simulink model "MicroMouse_RapidDevelopment"  (R2025a)
settings: Solver=FixedStepAuto  StartTime=0.0  StopTime=inf  RelTol=1e-3
PreLoadFcn:
  | addpath(genpath(pwd))
InitFcn:
  | addpath(genpath(pwd));
  | auto_program("MicroMouseProgramming_Code\build\release\MicroMouseProgramming")
  | STLINK_COMPORT = auto_COMPORT()
  | 
  | clearvars -except STLINK_COMPORT STLINK_DRIVE STM32_ODR
libraries: etargetslib x18, instrumentseriallib x2
settings Model: SILPILModeSetting=veronly  PacingRate=0.100000  ExtModeTrigDuration=10  Creator=JesseJabezArendse  LastModifiedBy=sanjannaidoo
settings SolverCC: ZeroCrossControl=EnableAll  EnableFixedStepZeroCrossing=on
settings OptimizationCC: ReuseModelBlockBuffer=off  PassReuseOutputArgsAs=Individual arguments  ZeroExternalMemoryAtStartup=off  ZeroInternalMemoryAtStartup=off  MaxStackSize=64  OptimizationLevel=level1  OptimizationCustomize=off  EfficientTunableParamExpr=on
settings DebuggingCC: SignalInfNanChecking=warning  ParameterPrecisionLossMsg=none  ParameterTunabilityLossMsg=error
settings HardwareCC: ProdBitPerPointer=32.0  ProdBitPerSizeT=32.0  ProdBitPerPtrDiffT=32.0  ProdLargestAtomicInteger=Long  ProdLargestAtomicFloat=Double  ProdWordSize=32.0  ProdLongLongMode=on  ProdHWDeviceType=ARM Compatible->ARM Cortex
settings ModelReferenceCC: EnableParallelModelReferenceBuilds=on
settings SFSimCC: SimParseCustomCode=off  MATLABDynamicMemAlloc=off  SimHardwareAcceleration=native
settings RTWCC: SystemTargetFile=ert.tlc  TemplateMakefile=ert_default_tmf  RTWUseSimCustomCode=on  Toolchain=GNU Tools for ARM Embedded Processors  BuildConfiguration=Specify  GPUComputeCapability=3.5  Description=Embedded Coder
settings CodeAppCC: ForceParamTrailComments=on  IgnoreCustomStorageClasses=off  OperatorAnnotations=on  SimulinkDataObjDesc=on  SFDataObjDesc=on  InsertBlockDesc=on
settings ERTTargetCC: ExtModeTransport=3.0  ExtModeStaticAllocSize=2000.0  InlinedParameterPlacement=Hierarchical  ERTCustomFileTemplate=example_file_process.tlc  DynamicArrayContainerType=coder::array  CodeReplacementLibrary=ARM Cortex-M  SupportContinuousTime=on
settings SimscapeCC: SimscapeLogDecimation=1  SimscapeLogDataHistory=5000

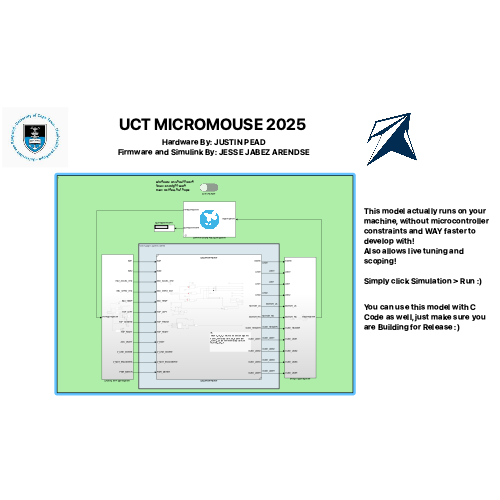
[thumbnail: Simulink's stored preview of the top-level diagram]
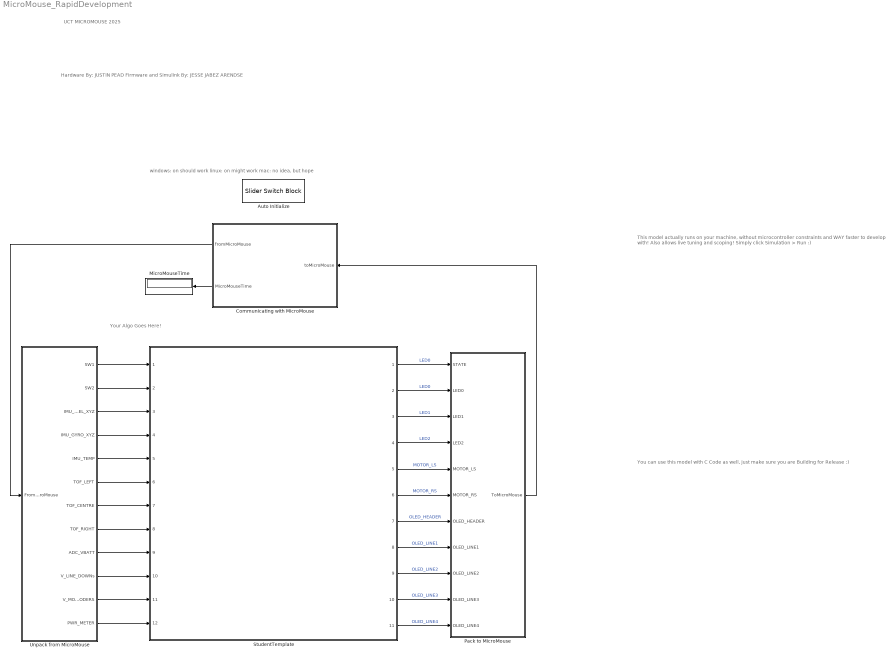
== system MicroMouse_RapidDevelopment ==
  note: windows: on should work
      | linux: on might work
      | mac: no idea, but hope
  note: Your Algo Goes Here!
  note: Hardware By: JUSTIN PEAD
      | Firmware and Simulink By: JESSE JABEZ ARENDSE
  note: UCT MICROMOUSE 2025
  note: This model actually runs on your machine, without microcontroller constraints and WAY faster to develop with!
      | Also allows live tuning and scoping!
      |
      | Simply click Simulation > Run :)
  note: You can use this model with C Code as well, just make sure you are Building for Release :)
  Auto Initialize : SliderSwitchBlock  LabelPosition=Hide
  Communicating with MicroMouse : Subsystem  mask{Auto_Initialize=0}
      mask prompts: Auto_Initialize "Automate Initialization?"
      mask TypeOptions Auto_Initialize: 1 | 0
      mask DialogControl Control1 Prompt: Block for communication between host machine and STM32L476 onboard MicroMouse
      mask Display: image('stm32_icon.png', [0,0,0,0,80,80]);
  MicroMouseTime : Display
      settings: Decimation=2
  Pack to MicroMouse : Subsystem
  StudentTemplate : Subsystem  ReferencedSubsystem=StudentTemplate
  Unpack from MicroMouse : Subsystem
  wires:
  Communicating with MicroMouse/2(MicroMouseTime) -> MicroMouseTime/1
  Pack to MicroMouse/1(ToMicroMouse) -> Communicating with MicroMouse/1(toMicroMouse)
  Communicating with MicroMouse/1(fromMicroMouse) -> Unpack from MicroMouse/1(FromMicroMouse)
  Unpack from MicroMouse/1(SW1) -> StudentTemplate/1
  Unpack from MicroMouse/2(SW2) -> StudentTemplate/2
  Unpack from MicroMouse/3(IMU_ACCEL_XYZ) -> StudentTemplate/3
  Unpack from MicroMouse/4(IMU_GYRO_XYZ) -> StudentTemplate/4
  Unpack from MicroMouse/5(IMU_TEMP) -> StudentTemplate/5
  Unpack from MicroMouse/6(TOF_LEFT) -> StudentTemplate/6
  Unpack from MicroMouse/7(TOF_CENTRE) -> StudentTemplate/7
  Unpack from MicroMouse/8(TOF_RIGHT) -> StudentTemplate/8
  Unpack from MicroMouse/9(ADC_VBATT) -> StudentTemplate/9
  Unpack from MicroMouse/10(V_LINE_DOWNs) -> StudentTemplate/10
  Unpack from MicroMouse/11(V_MOT_ENCODERS) -> StudentTemplate/11
  StudentTemplate/2 -> Pack to MicroMouse/2(LED0)  "LED0"
  StudentTemplate/3 -> Pack to MicroMouse/3(LED1)  "LED1"
  StudentTemplate/4 -> Pack to MicroMouse/4(LED2)  "LED2"
  StudentTemplate/5 -> Pack to MicroMouse/5(MOTOR_LS)  "MOTOR_LS"
  StudentTemplate/6 -> Pack to MicroMouse/6(MOTOR_RS)  "MOTOR_RS"
  StudentTemplate/7 -> Pack to MicroMouse/7(OLED_HEADER)  "OLED_HEADER"
  StudentTemplate/8 -> Pack to MicroMouse/8(OLED_LINE1)  "OLED_LINE1"
  StudentTemplate/9 -> Pack to MicroMouse/9(OLED_LINE2)  "OLED_LINE2"
  StudentTemplate/10 -> Pack to MicroMouse/10(OLED_LINE3)  "OLED_LINE3"
  StudentTemplate/11 -> Pack to MicroMouse/11(OLED_LINE4)  "OLED_LINE4"
  Unpack from MicroMouse/12(PWR_METER) -> StudentTemplate/12
  StudentTemplate/1 -> Pack to MicroMouse/1(STATE)  "LED0"

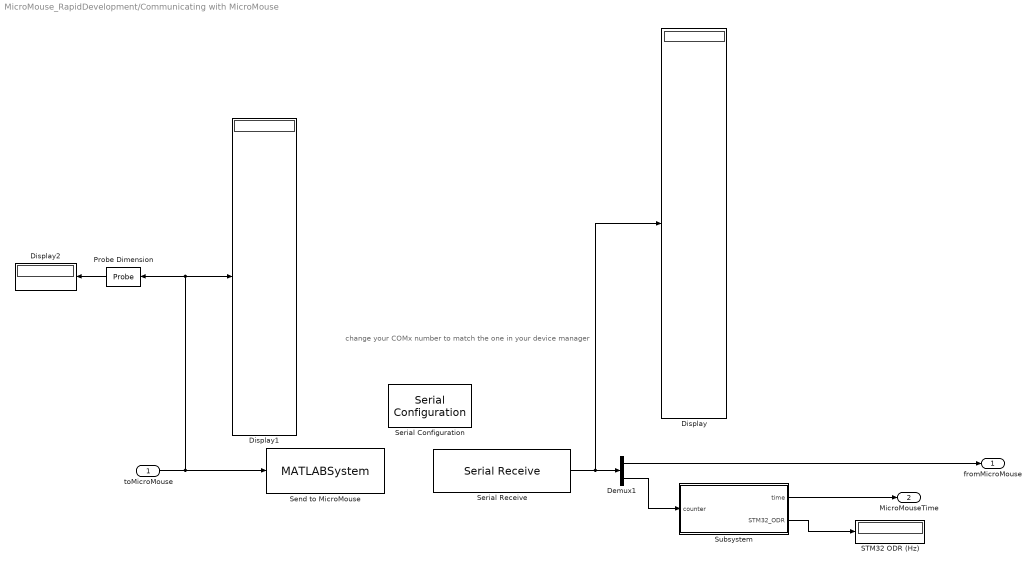
== system MicroMouse_RapidDevelopment/Communicating with MicroMouse ==
  note: change your COMx number to match the one in your device manager
  toMicroMouse : Inport
  Demux1 : Demux  Outputs=[29 1]
  Display : Display
  Display1 : Display
  Display2 : Display
  Probe Dimension : Probe  ProbeWidth=off  ProbeSampleTime=off  ProbeComplexSignal=off  ProbeSignalDimensions=on
  STM32 ODR (Hz) : Display
  Send to MicroMouse : MATLABSystem  System=CustomSerialSend  PortSel=STLINK_COMPORT  Header='J_A'  Terminator=Custom terminator  CustomTerminator='A_J'  ComPort=STLINK_COMPORT  EnableBlockingMode=off  SimulateUsing=Interpreted execution
      mask Type: CustomSerialSend
  Serial Configuration : instrumentseriallib/Serial Configuration  Priority=-200000  PortSel=STLINK_COMPORT  Port=STLINK_COMPORT  ComPort=STLINK_COMPORT  BaudRate=1843200  DataBits=8  Parity=none  StopBits=1  ByteOrder=little-endian  FlowControl=none  Timeout=1/100  SimulateUsing=Interpreted execution  BlockInModel=on  aMode=1
      settings: LibrarySourceBlock=embeddedtargetslib/Host Communication/Serial Configuration
  Serial Receive : instrumentseriallib/Serial Receive  Priority=1  PortSel=STLINK_COMPORT  Port=STLINK_COMPORT  ComPort=STLINK_COMPORT  DataType=single  SaveDataType=uint8  ToggleHeader=on  Header='J_A'  ToggleDataSize=on  DataSize="[1 2 + 3 + 3 + 1 + 4*3 + 5  + 1 + 3]"  ToggleTerminator=off  Terminator=Custom terminator  CustomTerminator='A_J'  InputFormat=Column major  EnableBlockingMode=on  ActionDataUnavailable=Output last received value  ActionWhenDataUnavailable=Output last received value  CustomValue=0  SampleTime=1/100  SimulateUsing=Interpreted execution  BlockInModel=on  aMode=1
      settings: LibrarySourceBlock=embeddedtargetslib/Host Communication/Serial Receive
  Subsystem : Subsystem
  fromMicroMouse : Outport
  MicroMouseTime : Outport  Port=2
  wires:
  Subsystem/2(STM32_ODR) -> STM32 ODR (Hz)/1
  Serial Receive/1 -> Demux1/1, Display/1
  toMicroMouse/1 -> Send to MicroMouse/1, Probe Dimension/1, Display1/1
  Subsystem/1(time) -> MicroMouseTime/1
  Demux1/2 -> Subsystem/1(counter)
  Demux1/1 -> fromMicroMouse/1
  Probe Dimension/1 -> Display2/1

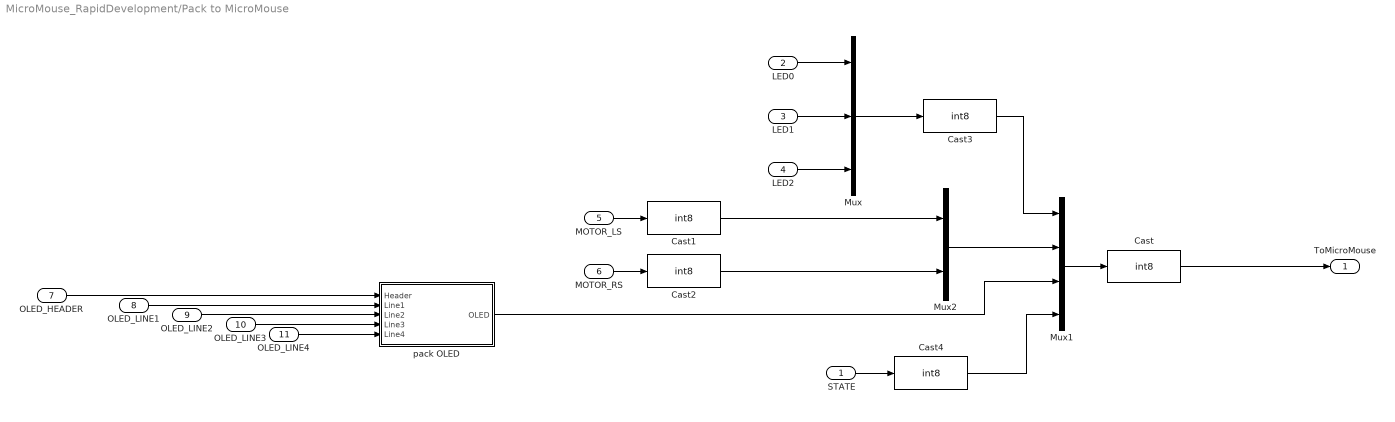
== system MicroMouse_RapidDevelopment/Pack to MicroMouse ==
  STATE : Inport
  LED0 : Inport  Port=2
  LED1 : Inport  Port=3
  LED2 : Inport  Port=4
  MOTOR_LS : Inport  Port=5
  MOTOR_RS : Inport  Port=6
  OLED_HEADER : Inport  Port=7  OutDataTypeStr=string
  OLED_LINE1 : Inport  Port=8  OutDataTypeStr=string
  OLED_LINE2 : Inport  Port=9  OutDataTypeStr=string
  OLED_LINE3 : Inport  Port=10  OutDataTypeStr=string
  OLED_LINE4 : Inport  Port=11  OutDataTypeStr=string
  Cast{,1..4} (5 alike) : DataTypeConversion  OutDataTypeStr=int8  SaturateOnIntegerOverflow=off  RndMeth=Floor
  Mux : Mux  Inputs=3
  Mux1 : Mux
  Mux2 : Mux  Inputs=2
  pack OLED : Subsystem
  ToMicroMouse : Outport
  wires:
  LED0/1 -> Mux/1
  Mux/1 -> Cast3/1
  LED1/1 -> Mux/2
  Cast3/1 -> Mux1/1
  LED2/1 -> Mux/3
  MOTOR_LS/1 -> Cast1/1
  MOTOR_RS/1 -> Cast2/1
  Mux2/1 -> Mux1/2
  pack OLED/1(OLED) -> Mux1/3
  Mux1/1 -> Cast/1
  Cast/1 -> ToMicroMouse/1
  OLED_HEADER/1 -> pack OLED/1(Header)
  OLED_LINE1/1 -> pack OLED/2(Line1)
  OLED_LINE2/1 -> pack OLED/3(Line2)
  OLED_LINE3/1 -> pack OLED/4(Line3)
  OLED_LINE4/1 -> pack OLED/5(Line4)
  Cast1/1 -> Mux2/1
  Cast2/1 -> Mux2/2
  STATE/1 -> Cast4/1
  Cast4/1 -> Mux1/4

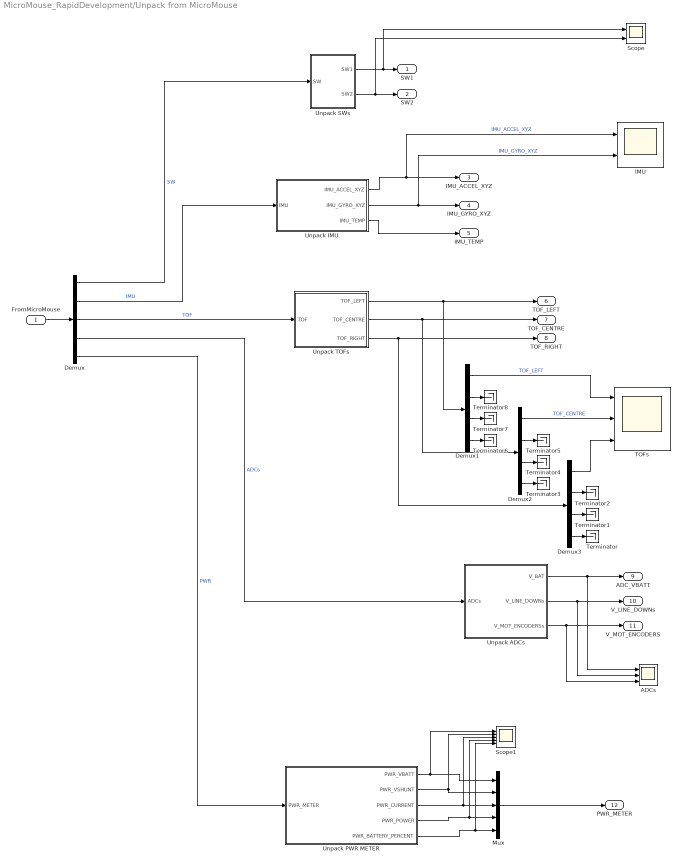
== system MicroMouse_RapidDevelopment/Unpack from MicroMouse ==
  FromMicroMouse : Inport
  ADCs : Scope  NumInputPorts=3
      settings: ActiveDisplayYMinimum=3.13868  ActiveDisplayYMaximum=3.14
  Demux : Demux  Outputs=[2 7 3*4 5 3]
  Demux1 : Demux
  Demux2 : Demux
  Demux3 : Demux
  IMU : Scope  NumInputPorts=2
      settings: ActiveDisplayYMinimum=-196.12162  ActiveDisplayYMaximum=196.12642
  Mux : Mux  Inputs=5
  Scope : Scope  NumInputPorts=2
      settings: ActiveDisplayYMinimum=0.9  ActiveDisplayYMaximum=1.1
  Scope1 : Scope  NumInputPorts=5
      settings: ActiveDisplayYMinimum=864.875  ActiveDisplayYMaximum=30696.125  DataLoggingVariableName=ScopeData2
  TOFs : Scope  NumInputPorts=3
      settings: ActiveDisplayYMinimum=0.02013  ActiveDisplayYMaximum=0.44888
  Terminator{,1..8} (9 alike) : Terminator
  Unpack ADCs : Subsystem
  Unpack IMU : Subsystem
  Unpack PWR METER : Subsystem
  Unpack SWs : Subsystem
  Unpack TOFs : Subsystem
  SW1 : Outport
  SW2 : Outport  Port=2
  IMU_ACCEL_XYZ : Outport  Port=3
  IMU_GYRO_XYZ : Outport  Port=4
  IMU_TEMP : Outport  Port=5
  TOF_LEFT : Outport  Port=6
  TOF_CENTRE : Outport  Port=7
  TOF_RIGHT : Outport  Port=8
  ADC_VBATT : Outport  Port=9
  V_LINE_DOWNs : Outport  Port=10
  V_MOT_ENCODERS : Outport  Port=11
  PWR_METER : Outport  Port=12
  wires:
  Unpack IMU/2(IMU_GYRO_XYZ) -> IMU/2, IMU_GYRO_XYZ/1  "IMU_GYRO_XYZ"
  Unpack IMU/1(IMU_ACCEL_XYZ) -> IMU/1, IMU_ACCEL_XYZ/1  "IMU_ACCEL_XYZ"
  Demux/1 -> Unpack SWs/1(SW)  "SW"
  FromMicroMouse/1 -> Demux/1
  Demux/2 -> Unpack IMU/1(IMU)  "IMU"
  Demux/3 -> Unpack TOFs/1(TOF)  "TOF"
  Demux/4 -> Unpack ADCs/1(ADCs)  "ADCs"
  Demux1/1 -> TOFs/1  "TOF_LEFT"
  Unpack SWs/1(SW1) -> Scope/1, SW1/1
  Unpack SWs/2(SW2) -> Scope/2, SW2/1
  Unpack IMU/3(IMU_TEMP) -> IMU_TEMP/1
  Unpack TOFs/1(TOF_LEFT) -> TOF_LEFT/1, Demux1/1
  Unpack TOFs/3(TOF_RIGHT) -> TOF_RIGHT/1, Demux3/1
  Unpack TOFs/2(TOF_CENTRE) -> TOF_CENTRE/1, Demux2/1
  Unpack ADCs/1(V_BAT) -> ADC_VBATT/1, ADCs/1
  Unpack ADCs/2(V_LINE_DOWNs) -> V_LINE_DOWNs/1, ADCs/2
  Unpack ADCs/3(V_MOT_ENCODERSs) -> V_MOT_ENCODERS/1, ADCs/3
  Demux1/3 -> Terminator7/1
  Demux1/2 -> Terminator8/1
  Demux1/4 -> Terminator6/1
  Demux2/1 -> TOFs/2  "TOF_CENTRE"
  Demux2/3 -> Terminator4/1
  Demux2/2 -> Terminator5/1
  Demux2/4 -> Terminator3/1
  Demux3/1 -> TOFs/3
  Demux3/3 -> Terminator1/1
  Demux3/2 -> Terminator2/1
  Demux3/4 -> Terminator/1
  Demux/5 -> Unpack PWR METER/1(PWR_METER)  "PWR"
  Unpack PWR METER/1(PWR_VBATT) -> Scope1/1, Mux/1
  Unpack PWR METER/2(PWR_VSHUNT) -> Mux/2, Scope1/2
  Unpack PWR METER/3(PWR_CURRENT) -> Mux/3, Scope1/3
  Unpack PWR METER/4(PWR_POWER) -> Mux/4, Scope1/4
  Unpack PWR METER/5(PWR_BATTERY_PERCENT) -> Scope1/5, Mux/5
  Mux/1 -> PWR_METER/1

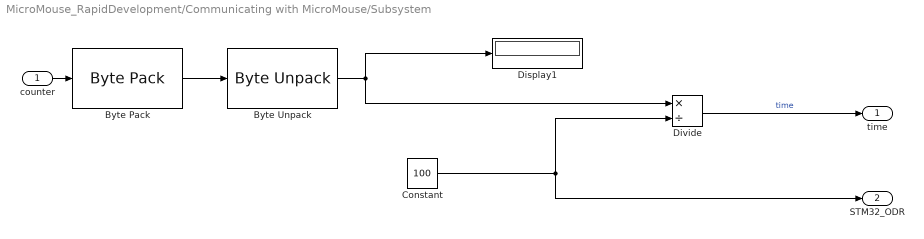
== system MicroMouse_RapidDevelopment/Communicating with MicroMouse/Subsystem ==
  counter : Inport
  Byte Pack : etargetslib/Byte Pack  datatypes={'single'}  byteAlign=1
  Byte Unpack : etargetslib/Byte Unpack  dimensions={[1]}  datatypes={'uint32'}  byteAlign=1
      settings: LibrarySourceBlock=embeddedtargetslib/Host Communication/Byte Unpack
  Constant : Constant  Value=100
  Display1 : Display
  Divide : Product  Inputs=*/
  time : Outport
  STM32_ODR : Outport  Port=2
  wires:
  counter/1 -> Byte Pack/1
  Divide/1 -> time/1  "time"
  Constant/1 -> STM32_ODR/1, Divide/2
  Byte Unpack/1 -> Divide/1, Display1/1
  Byte Pack/1 -> Byte Unpack/1

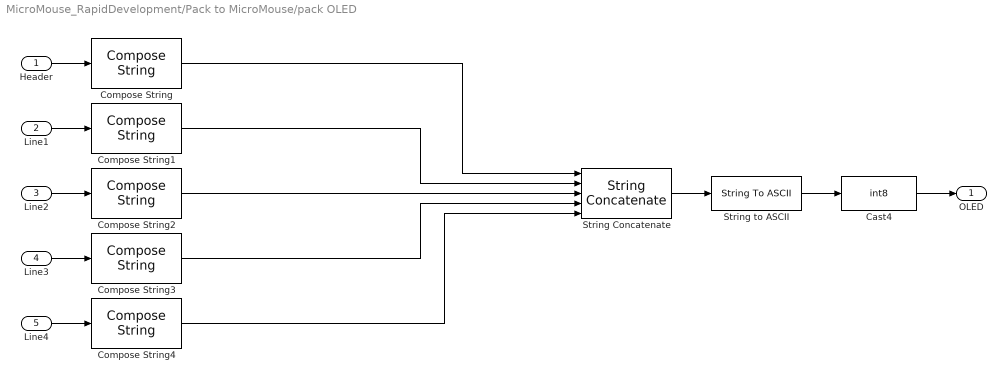
== system MicroMouse_RapidDevelopment/Pack to MicroMouse/pack OLED ==
  Header : Inport  PortDimensions=1
  Line1 : Inport  Port=2
  Line2 : Inport  Port=3
  Line3 : Inport  Port=4
  Line4 : Inport  Port=5
  Cast4 : DataTypeConversion  OutDataTypeStr=int8  SaturateOnIntegerOverflow=off  RndMeth=Floor
  Compose String{,1..4} (5 alike) : ComposeString  Format="\"%-18s\""
  String Concatenate : StringConcatenate  Inputs=5
  String to ASCII : StringToASCII  OutputVectorSize=18*5
  OLED : Outport
  wires:
  Header/1 -> Compose String/1
  Line1/1 -> Compose String1/1
  Line2/1 -> Compose String2/1
  Compose String1/1 -> String Concatenate/2
  Line3/1 -> Compose String3/1
  Line4/1 -> Compose String4/1
  Compose String/1 -> String Concatenate/1
  Compose String2/1 -> String Concatenate/3
  Compose String3/1 -> String Concatenate/4
  Compose String4/1 -> String Concatenate/5
  String Concatenate/1 -> String to ASCII/1
  String to ASCII/1 -> Cast4/1
  Cast4/1 -> OLED/1

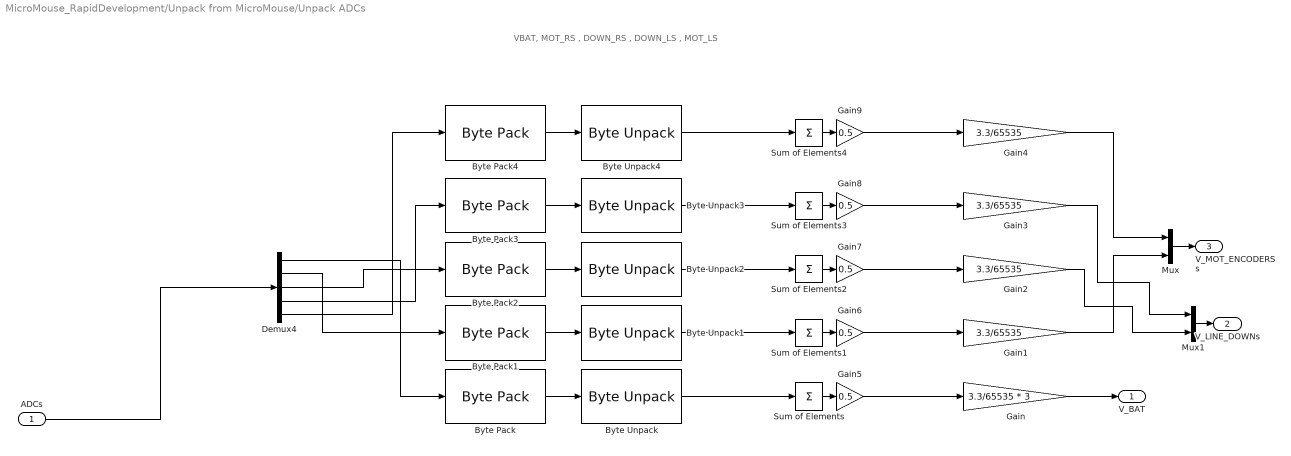
== system MicroMouse_RapidDevelopment/Unpack from MicroMouse/Unpack ADCs ==
  note: VBAT, MOT_RS , DOWN_RS , DOWN_LS , MOT_LS
  ADCs : Inport
  Byte Pack{,1..4} (5 alike) : etargetslib/Byte Pack  datatypes={'single'}  byteAlign=1
  Byte Unpack{,1..4} (5 alike) : etargetslib/Byte Unpack  dimensions={[2]}  datatypes={'uint16'}  byteAlign=1
      settings: LibrarySourceBlock=embeddedtargetslib/Host Communication/Byte Unpack
  Demux4 : Demux  Outputs=5
  Gain : Gain  Gain=3.3/65535 * 3
  Gain{1..4} (4 alike) : Gain  Gain=3.3/65535
  Gain{5..9} (5 alike) : Gain  Gain=0.5
  Mux : Mux  Inputs=2
  Mux1 : Mux  Inputs=2
  Sum of Elements{,1..4} (5 alike) : Sum  Inputs=+
  V_BAT : Outport
  V_LINE_DOWNs : Outport  Port=2
  V_MOT_ENCODERSs : Outport  Port=3
  wires:
  Gain8/1 -> Gain3/1
  Byte Pack/1 -> Byte Unpack/1
  Demux4/1 -> Byte Pack/1
  Gain9/1 -> Gain4/1
  Sum of Elements4/1 -> Gain9/1
  Gain3/1 -> Mux1/1
  Gain4/1 -> Mux/1
  Sum of Elements3/1 -> Gain8/1
  Mux/1 -> V_MOT_ENCODERSs/1
  Byte Unpack3/1 -> Sum of Elements3/1
  Demux4/3 -> Byte Pack2/1
  Demux4/5 -> Byte Pack4/1
  Byte Pack4/1 -> Byte Unpack4/1
  Byte Unpack4/1 -> Sum of Elements4/1
  Sum of Elements1/1 -> Gain6/1
  Gain7/1 -> Gain2/1
  Gain5/1 -> Gain/1
  Byte Pack3/1 -> Byte Unpack3/1
  Demux4/4 -> Byte Pack3/1
  Gain/1 -> V_BAT/1
  Demux4/2 -> Byte Pack1/1
  Byte Unpack/1 -> Sum of Elements/1
  Gain1/1 -> Mux/2
  Byte Unpack1/1 -> Sum of Elements1/1
  Sum of Elements/1 -> Gain5/1
  Mux1/1 -> V_LINE_DOWNs/1
  ADCs/1 -> Demux4/1
  Gain2/1 -> Mux1/2
  Byte Unpack2/1 -> Sum of Elements2/1
  Gain6/1 -> Gain1/1
  Byte Pack2/1 -> Byte Unpack2/1
  Byte Pack1/1 -> Byte Unpack1/1
  Sum of Elements2/1 -> Gain7/1

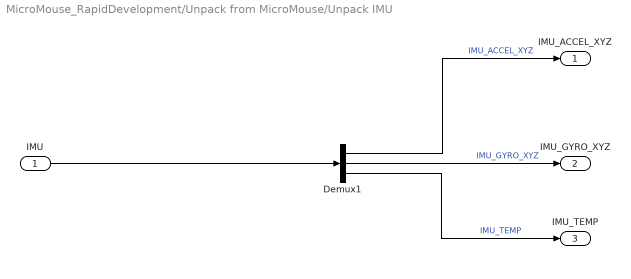
== system MicroMouse_RapidDevelopment/Unpack from MicroMouse/Unpack IMU ==
  IMU : Inport
  Demux1 : Demux  Outputs=[3 3 1]
  IMU_ACCEL_XYZ : Outport
  IMU_GYRO_XYZ : Outport  Port=2
  IMU_TEMP : Outport  Port=3
  wires:
  IMU/1 -> Demux1/1
  Demux1/2 -> IMU_GYRO_XYZ/1  "IMU_GYRO_XYZ"
  Demux1/1 -> IMU_ACCEL_XYZ/1  "IMU_ACCEL_XYZ"
  Demux1/3 -> IMU_TEMP/1  "IMU_TEMP"

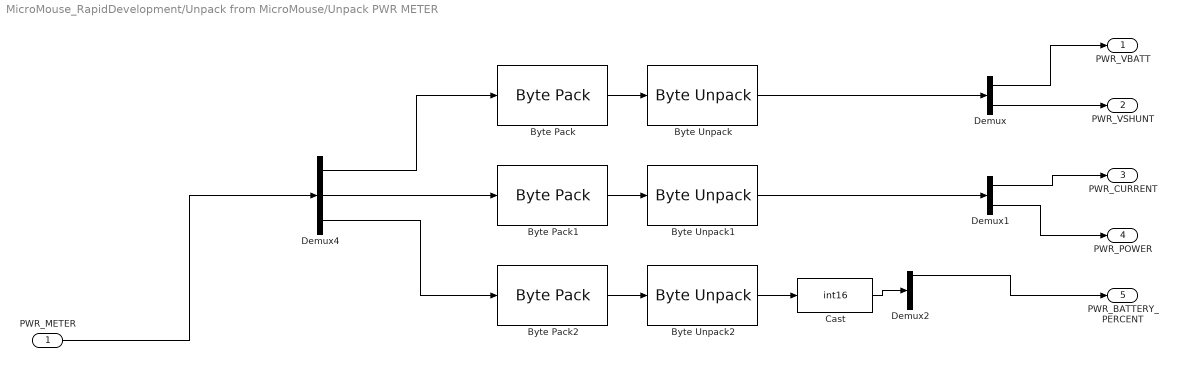
== system MicroMouse_RapidDevelopment/Unpack from MicroMouse/Unpack PWR METER ==
  PWR_METER : Inport
  Byte Pack : etargetslib/Byte Pack  datatypes={'single'}  byteAlign=1
  Byte Pack1 : etargetslib/Byte Pack  datatypes={'single'}  byteAlign=1
  Byte Pack2 : etargetslib/Byte Pack  datatypes={'single'}  byteAlign=1
  Byte Unpack : etargetslib/Byte Unpack  dimensions={[2]}  datatypes={'int16'}  byteAlign=1
  Byte Unpack1 : etargetslib/Byte Unpack  dimensions={[2]}  datatypes={'int16'}  byteAlign=1
  Byte Unpack2 : etargetslib/Byte Unpack  dimensions={[4]}  datatypes={'uint8'}  byteAlign=1
  Cast : DataTypeConversion  OutDataTypeStr=int16  SaturateOnIntegerOverflow=off  RndMeth=Floor
  Demux : Demux  Outputs=2
  Demux1 : Demux  Outputs=2
  Demux2 : Demux
  Demux4 : Demux  Outputs=3
  PWR_VBATT : Outport
  PWR_VSHUNT : Outport  Port=2
  PWR_CURRENT : Outport  Port=3
  PWR_POWER : Outport  Port=4
  PWR_BATTERY_PERCENT : Outport  Port=5
  wires:
  Byte Pack1/1 -> Byte Unpack1/1
  Byte Pack2/1 -> Byte Unpack2/1
  PWR_METER/1 -> Demux4/1
  Demux4/2 -> Byte Pack1/1
  Demux2/1 -> PWR_BATTERY_PERCENT/1
  Demux4/3 -> Byte Pack2/1
  Demux4/1 -> Byte Pack/1
  Byte Pack/1 -> Byte Unpack/1
  Demux/1 -> PWR_VBATT/1
  Demux/2 -> PWR_VSHUNT/1
  Demux1/2 -> PWR_POWER/1
  Demux1/1 -> PWR_CURRENT/1
  Byte Unpack/1 -> Demux/1
  Byte Unpack1/1 -> Demux1/1
  Byte Unpack2/1 -> Cast/1
  Cast/1 -> Demux2/1

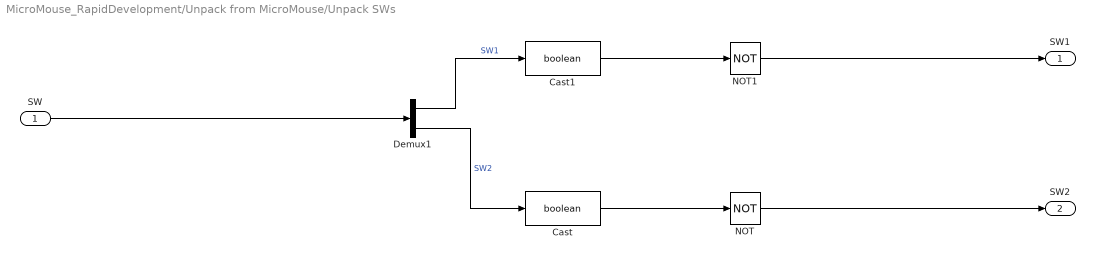
== system MicroMouse_RapidDevelopment/Unpack from MicroMouse/Unpack SWs ==
  SW : Inport
  Cast : DataTypeConversion  OutDataTypeStr=boolean  SaturateOnIntegerOverflow=off  RndMeth=Floor
  Cast1 : DataTypeConversion  OutDataTypeStr=boolean  SaturateOnIntegerOverflow=off  RndMeth=Floor
  Demux1 : Demux  Outputs=2
  NOT : Logic  Operator=NOT  IconShape=distinctive  AllPortsSameDT=off  OutDataTypeStr=boolean
  NOT1 : Logic  Operator=NOT  IconShape=distinctive  AllPortsSameDT=off  OutDataTypeStr=boolean
  SW1 : Outport
  SW2 : Outport  Port=2
  wires:
  Demux1/1 -> Cast1/1  "SW1"
  Demux1/2 -> Cast/1  "SW2"
  SW/1 -> Demux1/1
  Cast/1 -> NOT/1
  Cast1/1 -> NOT1/1
  NOT/1 -> SW2/1
  NOT1/1 -> SW1/1

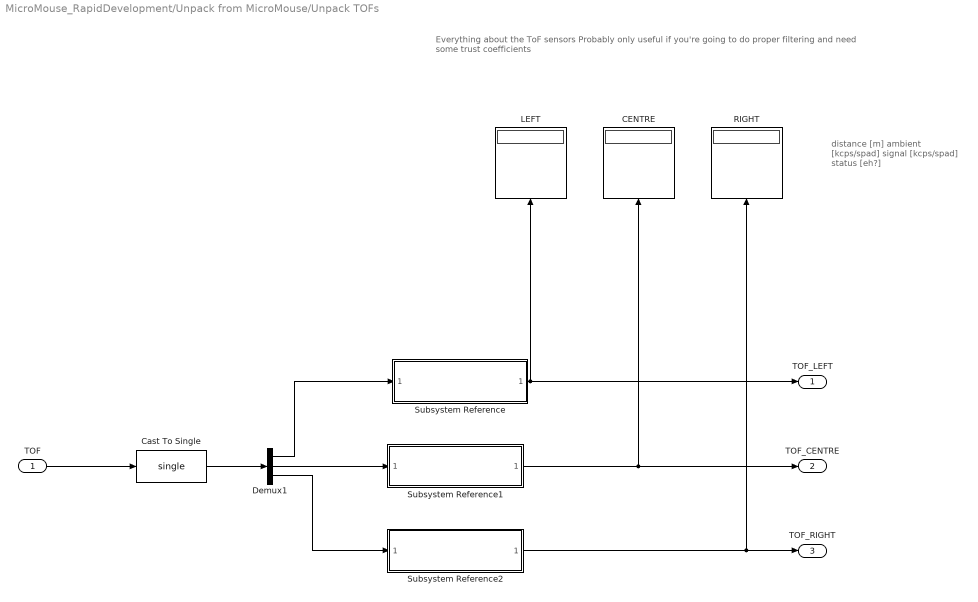
== system MicroMouse_RapidDevelopment/Unpack from MicroMouse/Unpack TOFs ==
  note: Everything about the ToF sensors
      | Probably only useful if you're going to do proper filtering and need some trust coefficients
  note: distance [m]
      | ambient [kcps/spad]
      | signal [kcps/spad]
      | status [eh?]
  TOF : Inport
  CENTRE : Display
  Cast To Single : DataTypeConversion  OutDataTypeStr=single  SaturateOnIntegerOverflow=off  RndMeth=Floor
  Demux1 : Demux  Outputs=[4 4 4]
  LEFT : Display
  RIGHT : Display
  Subsystem Reference : Subsystem  ReferencedSubsystem=unpack_ToF
  Subsystem Reference1 : Subsystem  ReferencedSubsystem=unpack_ToF
  Subsystem Reference2 : Subsystem  ReferencedSubsystem=unpack_ToF
  TOF_LEFT : Outport
  TOF_CENTRE : Outport  Port=2
  TOF_RIGHT : Outport  Port=3
  wires:
  TOF/1 -> Cast To Single/1
  Demux1/2 -> Subsystem Reference1/1
  Demux1/1 -> Subsystem Reference/1
  Cast To Single/1 -> Demux1/1
  Demux1/3 -> Subsystem Reference2/1
  Subsystem Reference/1 -> TOF_LEFT/1, LEFT/1
  Subsystem Reference2/1 -> TOF_RIGHT/1, RIGHT/1
  Subsystem Reference1/1 -> TOF_CENTRE/1, CENTRE/1
